simulink model "Adaptive_NonLinear_Control_For_Active_Suspension"  (R2023b)
settings: Solver=VariableStepAuto  StartTime=0.0  StopTime=40.0  MaxStep=1e-4  RelTol=1e-3
values from neighbouring files (symbols this model uses):
  A = [0 1 0 0; -(kc_sse/mc_sse) -(cc_sse/mc_sse) (kc_sse/mc_sse) (cc_sse/mc_sse); 0 0 0 1; (kc_sse/mw_sse) (cc_sse/mw_sse) -((kc_sse + kw_sse)/mw_sse) -(cc_sse/mw_sse)]    [Active_Suspension_1.m]    (also in Active_Suspension_Control.m = [ 0 1 0 0; [-k_car -c_car k_car c_car]/m_car ; 0 0 0 1; [k_c; Active_With_Robust_Road.m; Extras.m; Robust_Active_Suspension_Control.m = [ 0 1 0 0; [-k_car -c_car k_car c_car]/m_car ; 0 0 0 1; [k_c)
  B = [0 0; (1/mc_sse) 0; 0 0; -(1/mw_sse) (kw_sse/ mw_sse)]    [Active_Suspension_1.m]    (also in Active_Suspension_Control.m = [ 0 0; 0 1/m_car ; 0 0 ; [-1 k_wheel]/m_wheel]; Active_With_Robust_Road.m; Extras.m; Robust_Active_Suspension_Control.m = [ 0 0; 0 1e3/m_car ; 0 0 ; [k_wheel -1e3]/m_wheel])
  C = [1 0 0 0]    [Active_Suspension_1.m]    (also in Active_Suspension_Control.m; Active_With_Robust_Road.m; Extras.m; Robust_Active_Suspension_Control.m = [1 0 0 0; 1 0 -1 0; A(2,:)])
  cc_1 = 30    [Extras.m]
  D = [0 0]    [Active_Suspension_1.m]    (also in Active_Suspension_Control.m; Active_With_Robust_Road.m; Extras.m; Robust_Active_Suspension_Control.m = [0 0; 0 0; B(2,:)])
  kc_1 = 23    [Extras.m]
  kw_1 = 700    [Extras.m]
  mc_1 = 60    [Extras.m]
  mw_1 = 12    [Extras.m]
  u1 = [uc; ud]    [Robust_With_Adaptive_Road.m]
settings Model: Creator=hkurt  LastModifiedBy=hkurt

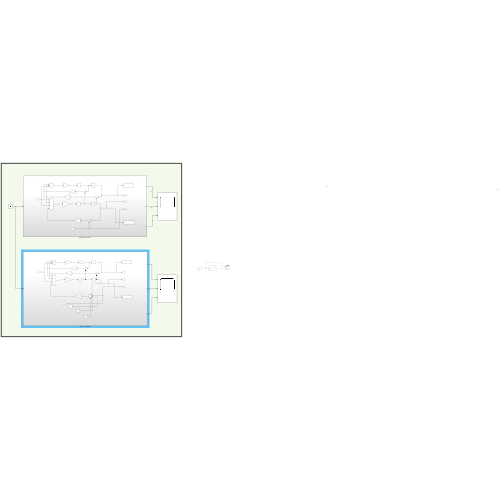
[thumbnail: Simulink's stored preview of the top-level diagram]
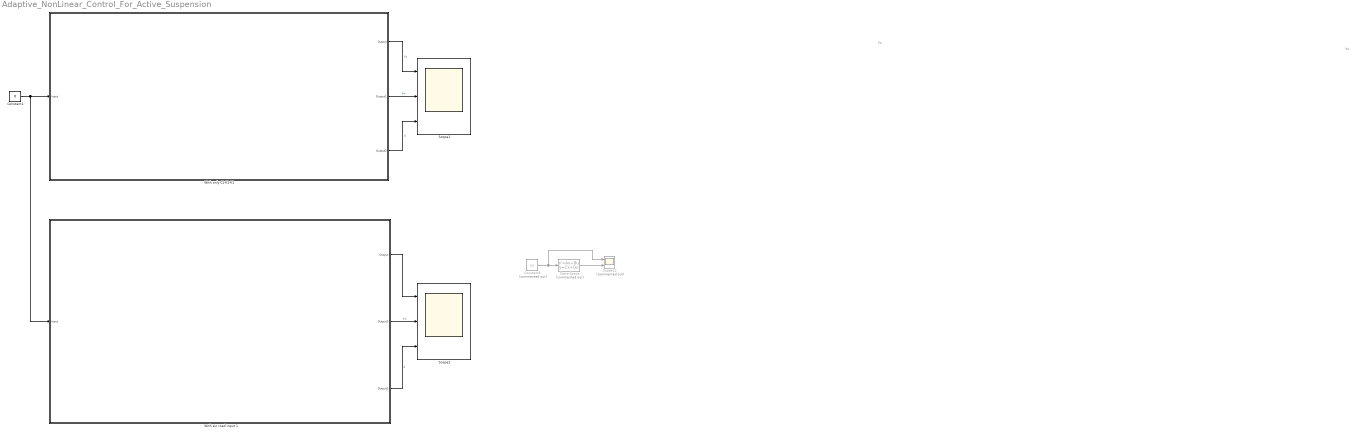
== system Adaptive_NonLinear_Control_For_Active_Suspension ==
  note: Yc
  note: Yc
  Constant1 : Constant  Value=0
  Constant6 : Constant  Commented=on  Value=u1
  Scope1 : Scope  NumInputPorts=3
  Scope12 : Scope  Commented=on  NumInputPorts=2
  Scope2 : Scope  NumInputPorts=3
  State-Space : StateSpace  Commented=on  A=A  B=B  C=C  D=D  InitialCondition=0
  With only C1-K1-K1 : Subsystem
  With sin road input 1 : Subsystem
  wires:
  Constant1/1 -> With only C1-K1-K1/1(Input), With sin road input 1/1(Input)
  With only C1-K1-K1/1(Output) -> Scope1/1  "Yc"
  With only C1-K1-K1/2(Output1) -> Scope1/2  "Yw"
  With only C1-K1-K1/3(Output2) -> Scope1/3  "X"
  With sin road input 1/3(Output2) -> Scope2/3  "X"
  With sin road input 1/2(Output1) -> Scope2/2  "Yw"
  With sin road input 1/1(Output) -> Scope2/1
  State-Space/1 -> Scope12/2
  Constant6/1 -> Scope12/1, State-Space/1

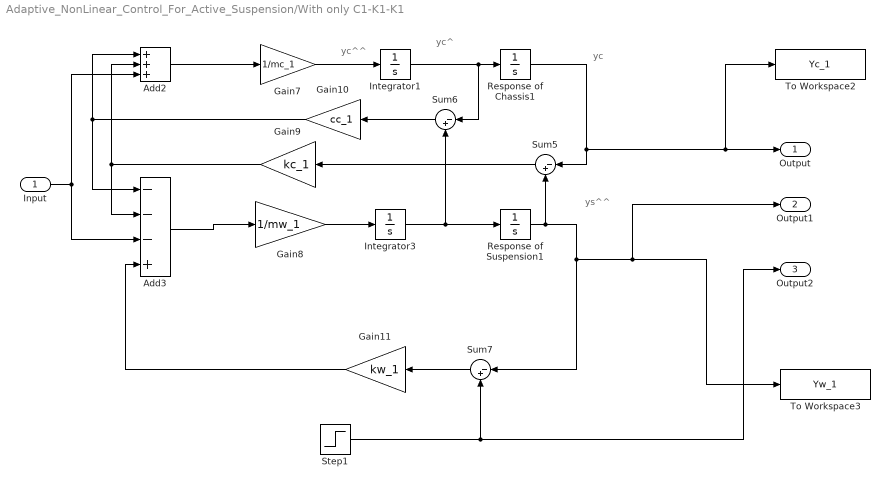
== system Adaptive_NonLinear_Control_For_Active_Suspension/With only C1-K1-K1 ==
  note: ys^^
  note: yc^^
  note: yc
  note: yc^
  Input : Inport
  Add2 : Sum  Inputs=+++
  Add3 : Sum  Inputs=---+
  Gain10 : Gain  Gain=cc_1
  Gain11 : Gain  Gain=kw_1
  Gain7 : Gain  Gain=1/mc_1
  Gain8 : Gain  Gain=1/mw_1
  Gain9 : Gain  Gain=kc_1
  Integrator1 : Integrator
  Integrator3 : Integrator
  Response of Chassis1 : Integrator
  Response of Suspension1 : Integrator
  Step1 : Step  After=30  SampleTime=0
  Sum5 : Sum  Inputs=|-+
  Sum6 : Sum  Inputs=|-+
  Sum7 : Sum  Inputs=|-+
  To Workspace2 : ToWorkspace  VariableName=Yc_1  SaveFormat=Timeseries  SampleTime=-1
  To Workspace3 : ToWorkspace  VariableName=Yw_1  SaveFormat=Timeseries  SampleTime=-1
  Output : Outport
  Output1 : Outport  Port=2
  Output2 : Outport  Port=3
  wires:
  Gain11/1 -> Add3/4
  Sum5/1 -> Gain9/1
  Add3/1 -> Gain8/1
  Response of Suspension1/1 -> Sum5/2, Sum7/1, Output1/1, To Workspace3/1
  Sum7/1 -> Gain11/1
  Integrator1/1 -> Sum6/1, Response of Chassis1/1
  Gain8/1 -> Integrator3/1
  Gain9/1 -> Add3/2, Add2/2
  Sum6/1 -> Gain10/1
  Response of Chassis1/1 -> Sum5/1, Output/1, To Workspace2/1
  Gain7/1 -> Integrator1/1
  Step1/1 -> Output2/1, Sum7/2
  Integrator3/1 -> Sum6/2, Response of Suspension1/1
  Add2/1 -> Gain7/1
  Gain10/1 -> Add3/1, Add2/1
  Input/1 -> Add2/3, Add3/3

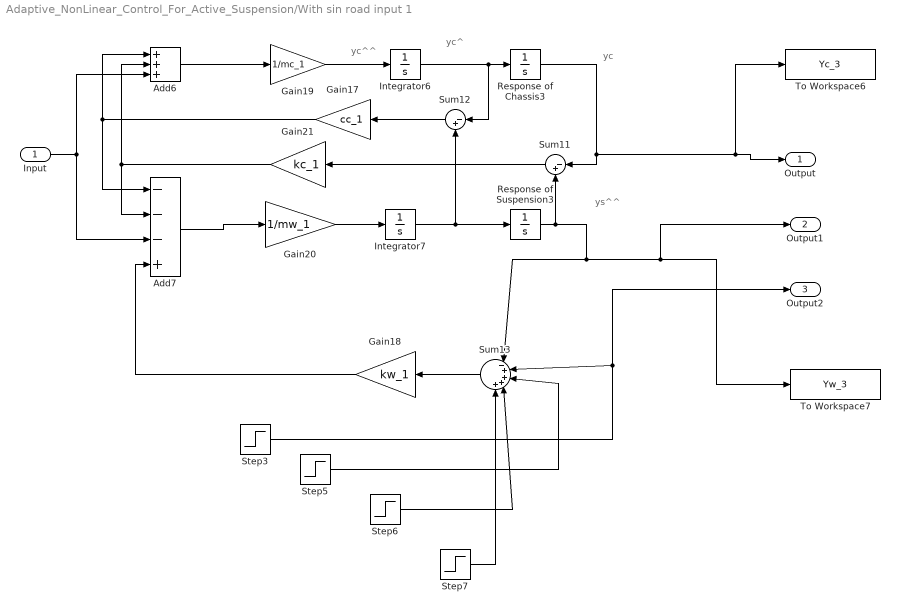
== system Adaptive_NonLinear_Control_For_Active_Suspension/With sin road input 1 ==
  note: yc^^
  note: yc^
  note: yc
  note: ys^^
  Input : Inport
  Add6 : Sum  Inputs=+++
  Add7 : Sum  Inputs=---+
  Gain17 : Gain  Gain=cc_1
  Gain18 : Gain  Gain=kw_1
  Gain19 : Gain  Gain=1/mc_1
  Gain20 : Gain  Gain=1/mw_1
  Gain21 : Gain  Gain=kc_1
  Integrator6 : Integrator
  Integrator7 : Integrator
  Response of Chassis3 : Integrator
  Response of Suspension3 : Integrator
  Step3 : Step  Time=5  After=10  SampleTime=0
  Step5 : Step  Time=10  After=20  SampleTime=0
  Step6 : Step  Time=15  After=-10  SampleTime=0
  Step7 : Step  Time=20  After=5  SampleTime=0
  Sum11 : Sum  Inputs=|-+
  Sum12 : Sum  Inputs=|-+
  Sum13 : Sum  Inputs=|-++++
  To Workspace6 : ToWorkspace  VariableName=Yc_3  SaveFormat=Timeseries  SampleTime=-1
  To Workspace7 : ToWorkspace  VariableName=Yw_3  SaveFormat=Timeseries  SampleTime=-1
  Output : Outport
  Output1 : Outport  Port=2
  Output2 : Outport  Port=3
  wires:
  Step7/1 -> Sum13/5
  Add6/1 -> Gain19/1
  Gain18/1 -> Add7/4
  Integrator6/1 -> Sum12/1, Response of Chassis3/1
  Sum12/1 -> Gain17/1
  Step3/1 -> Sum13/2, Output2/1
  Add7/1 -> Gain20/1
  Gain19/1 -> Integrator6/1
  Gain20/1 -> Integrator7/1
  Integrator7/1 -> Sum12/2, Response of Suspension3/1
  Response of Chassis3/1 -> Sum11/1, Output/1, To Workspace6/1
  Sum13/1 -> Gain18/1
  Response of Suspension3/1 -> Sum11/2, Sum13/1, Output1/1, To Workspace7/1
  Gain17/1 -> Add7/1, Add6/1
  Sum11/1 -> Gain21/1
  Step5/1 -> Sum13/3
  Step6/1 -> Sum13/4
  Gain21/1 -> Add7/2, Add6/2
  Input/1 -> Add7/3, Add6/3
